simulink model "testing"  (R2022a)
settings: Solver=VariableStepAuto  StartTime=0.0  StopTime=10.0  RelTol=1e-7
libraries: fuzblock x1
settings Model: Creator=sucho  LastModifiedBy=sucho

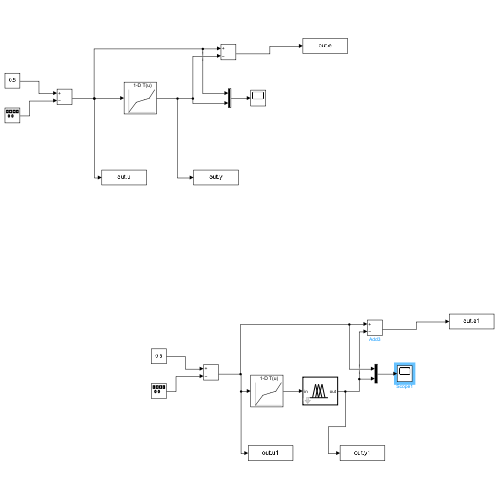
[thumbnail: Simulink's stored preview of the top-level diagram]
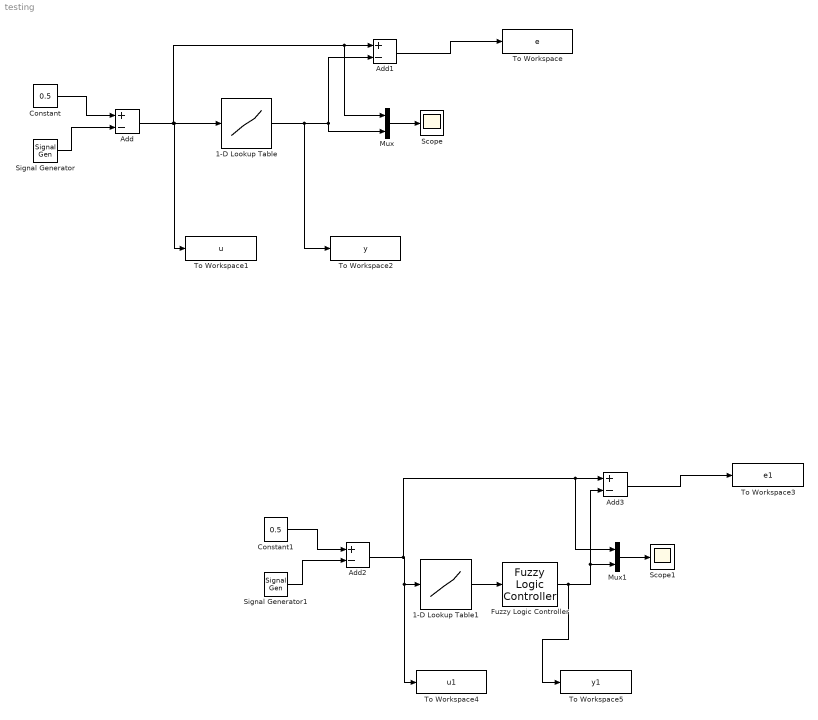
== system testing ==
  1-D Lookup Table : Lookup_n-D  NumberOfTableDimensions=1  BreakpointsForDimension1=[-0 0.3 0.6 0.8 1]  Table=[3 7 8 8.5 12]  InternalRulePriority=Speed  RndMeth=Simplest
  1-D Lookup Table1 : Lookup_n-D  NumberOfTableDimensions=1  BreakpointsForDimension1=[0 0.3 0.6 0.8 1]  Table=[3 7 8 8.5 12]  InternalRulePriority=Speed  RndMeth=Simplest
  Add{,1..3} (4 alike) : Sum  Inputs=+-
  Constant : Constant  Value=0.5
  Constant1 : Constant  Value=0.5
  Fuzzy Logic Controller : fuzblock/Fuzzy Logic  Controller  FIS=neko  OutputSampleNumber=101  DataType=double  FuzzifiedInputs=off  RuleFiringStrengths=off  RuleOutputs=off  AggregatedOutputs=off  SimulateUsing=Interpreted execution  OutOfRangeInputValueMessage=warning  NoRuleFiredMessage=warning  EmptyOutputFuzzySetMessage=warning
  Mux : Mux  Inputs=2
  Mux1 : Mux  Inputs=2
  Scope : Scope
  Scope1 : Scope
  Signal Generator : SignalGenerator  Amplitude=0.5  Units=rad/sec
  Signal Generator1 : SignalGenerator  Amplitude=0.5  Units=rad/sec
  To Workspace : ToWorkspace  VariableName=e  SaveFormat=Timeseries  SampleTime=0.1
  To Workspace1 : ToWorkspace  VariableName=u  SaveFormat=Timeseries  SampleTime=0.1
  To Workspace2 : ToWorkspace  VariableName=y  SaveFormat=Timeseries  SampleTime=0.1
      settings: Save2DSignal=2-D array (concatenate along first dimension)
  To Workspace3 : ToWorkspace  VariableName=e1  SaveFormat=Timeseries  SampleTime=0.1
  To Workspace4 : ToWorkspace  VariableName=u1  SaveFormat=Timeseries  SampleTime=0.1
  To Workspace5 : ToWorkspace  VariableName=y1  SaveFormat=Timeseries  SampleTime=0.1
      settings: Save2DSignal=2-D array (concatenate along first dimension)
  wires:
  Constant/1 -> Add/1
  Signal Generator/1 -> Add/2
  Add/1 -> Mux/1, Add1/1, To Workspace1/1, 1-D Lookup Table/1
  1-D Lookup Table/1 -> To Workspace2/1, Add1/2, Mux/2
  Mux/1 -> Scope/1
  Add1/1 -> To Workspace/1
  Mux1/1 -> Scope1/1
  Add2/1 -> Mux1/1, Add3/1, To Workspace4/1, 1-D Lookup Table1/1
  Constant1/1 -> Add2/1
  Add3/1 -> To Workspace3/1
  Signal Generator1/1 -> Add2/2
  1-D Lookup Table1/1 -> Fuzzy Logic Controller/1
  Fuzzy Logic Controller/1 -> To Workspace5/1, Add3/2, Mux1/2
